simulink model "models_diff_integr"  (R2017a)
settings: Solver=VariableStepAuto  StartTime=0.0  StopTime=Time  RelTol=1e-3
undefined symbols (not defined in the file or in its folder): coeff, coeff_integrator, ts
settings Model: FPTShortcutValueString='{{},{''BaselineRun'',1,1,1,''BaselineRun'','''',{},''M'',''D'',''''}}'  Creator=kavru  LastModifiedBy=kavru
settings DataIOCC: ReturnWorkspaceOutputs=on
settings DebuggingCC: SignalRangeChecking=warning  SFMachineParentedDataDiag=error
settings SFSimCC: SimUseLocalCustomCode=on
settings RTWCC: RTWUseLocalCustomCode=on

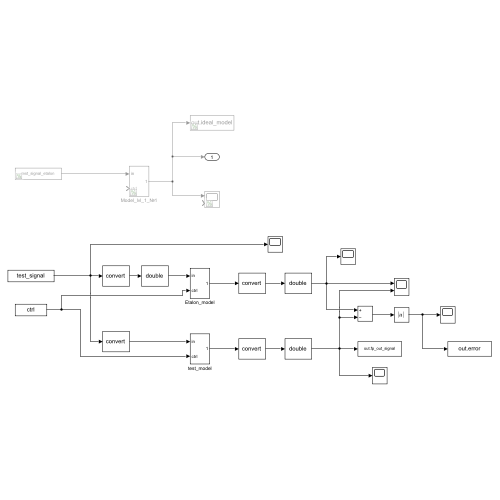
[thumbnail: Simulink's stored preview of the top-level diagram]
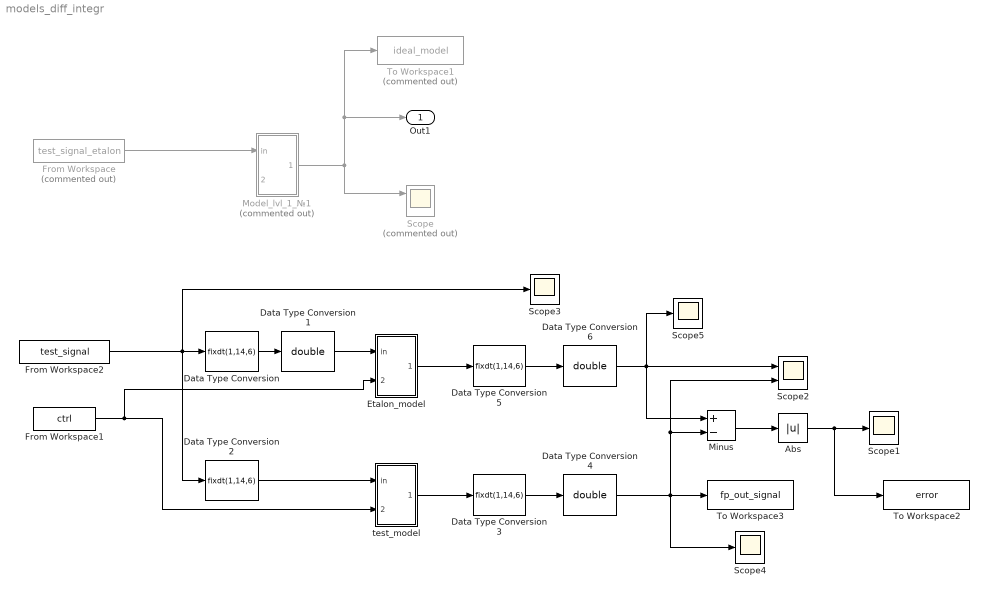
== system models_diff_integr ==
  Abs : Abs
  Data Type Conversion{,2..3,5} (4 alike) : DataTypeConversion  OutDataTypeStr=fixdt(1,14,6)  RndMeth=Nearest
  Data Type Conversion1 : DataTypeConversion  OutDataTypeStr=double
  Data Type Conversion4 : DataTypeConversion  OutDataTypeStr=double
  Data Type Conversion6 : DataTypeConversion  OutDataTypeStr=double
  Etalon_model : Subsystem
  From Workspace : FromWorkspace  Commented=on  VariableName=test_signal_etalon  OutDataTypeStr=double  SampleTime=ts
  From Workspace1 : FromWorkspace  VariableName=ctrl  SampleTime=ts
  From Workspace2 : FromWorkspace  VariableName=test_signal  OutDataTypeStr=double  SampleTime=ts
  Minus : Sum  Inputs=+-
  Model_lvl_1_№1 : Subsystem  Commented=on
  Scope : Scope  Commented=on  NumInputPorts=2
  Scope{1,3..5} (4 alike) : Scope
  Scope2 : Scope  NumInputPorts=2
  To Workspace1 : ToWorkspace  Commented=on  VariableName=ideal_model  SaveFormat=Timeseries  SampleTime=-1
  To Workspace2 : ToWorkspace  VariableName=error  SaveFormat=Timeseries  SampleTime=-1
  To Workspace3 : ToWorkspace  VariableName=fp_out_signal  SaveFormat=Timeseries  SampleTime=-1
  test_model : Subsystem
  Out1 : Outport
  wires:
  From Workspace/1 -> Model_lvl_1_№1/1(in)
  Model_lvl_1_№1/1(Out1) -> To Workspace1/1, Out1/1, Scope/1
  From Workspace2/1 -> Data Type Conversion2/1, Data Type Conversion/1, Scope3/1
  Minus/1 -> Abs/1
  Abs/1 -> Scope1/1, To Workspace2/1
  Data Type Conversion3/1 -> Data Type Conversion4/1
  Data Type Conversion4/1 -> To Workspace3/1, Minus/2, Scope2/2, Scope4/1
  Data Type Conversion6/1 -> Scope2/1, Minus/1, Scope5/1
  Data Type Conversion5/1 -> Data Type Conversion6/1
  From Workspace1/1 -> Etalon_model/2(ctrl), test_model/2(ctrl)
  test_model/1(Out1) -> Data Type Conversion3/1
  Etalon_model/1(Out1) -> Data Type Conversion5/1
  Data Type Conversion1/1 -> Etalon_model/1(in)
  Data Type Conversion2/1 -> test_model/1(in)
  Data Type Conversion/1 -> Data Type Conversion1/1

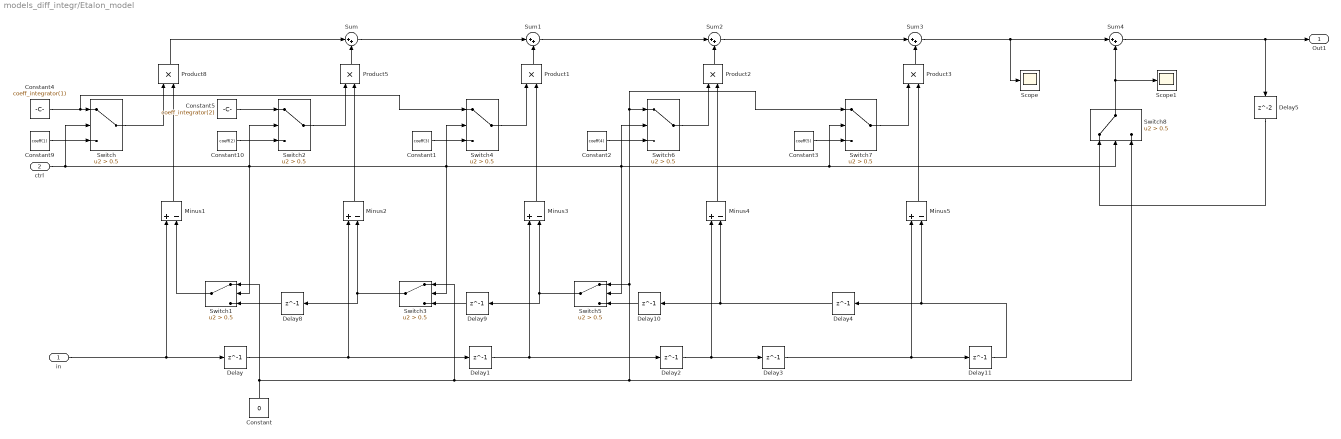
== system models_diff_integr/Etalon_model ==
  in : Inport
  ctrl : Inport  Port=2
  Constant : Constant  Value=0
  Constant1 : Constant  Value=coeff(3)
  Constant10 : Constant  Value=coeff(2)
  Constant2 : Constant  Value=coeff(4)
  Constant3 : Constant  Value=coeff(5)
  Constant4 : Constant  Value=coeff_integrator(1)
  Constant5 : Constant  Value=coeff_integrator(2)
  Constant9 : Constant  Value=coeff(1)
  Delay{,1..4,8..11} (9 alike) : Delay  DelayLength=1
  Delay5 : Delay
  Minus{1..5} (5 alike) : Sum  Inputs=+-  RndMeth=Nearest
  Product{1..3,5,8} (5 alike) : Product  RndMeth=Nearest
  Scope : Scope
  Scope1 : Scope
  Sum{,1..4} (5 alike) : Sum  Inputs=|++  RndMeth=Nearest
  Switch{,1..7} (8 alike) : Switch  Criteria=u2 > Threshold  Threshold=0.5
  Switch8 : Switch  Criteria=u2 > Threshold  Threshold=0.5  RndMeth=Nearest
  Out1 : Outport
  wires:
  Switch4/1 -> Product1/1
  Minus5/1 -> Product3/2
  Switch2/1 -> Product5/1
  Switch7/1 -> Product3/1
  Constant3/1 -> Switch7/3
  Sum1/1 -> Sum2/1
  Constant4/1 -> Switch4/1, Switch/1
  ctrl/1 -> Switch/2, Switch1/2, Switch7/2, Switch8/2, Switch6/2, Switch5/2, Switch3/2, Switch4/2, Switch2/2
  Minus4/1 -> Product2/2
  Constant10/1 -> Switch2/3
  Switch6/1 -> Product2/1
  Constant2/1 -> Switch6/3
  Sum4/1 -> Out1/1, Delay5/1
  Delay4/1 -> Minus4/2, Delay10/1
  Constant1/1 -> Switch4/3
  Delay/1 -> Delay1/1, Minus2/1
  Constant9/1 -> Switch/3
  Minus2/1 -> Product5/2
  Switch8/1 -> Scope1/1, Sum4/2
  Product5/1 -> Sum/2
  Product8/1 -> Sum/1
  Switch3/1 -> Delay8/1, Minus2/2
  Delay9/1 -> Switch3/3
  Sum3/1 -> Scope/1, Sum4/1
  Switch/1 -> Product8/1
  Constant/1 -> Switch1/1, Switch3/1, Switch6/1, Switch7/1, Switch5/1, Switch8/3
  Minus1/1 -> Product8/2
  Product3/1 -> Sum3/2
  Product1/1 -> Sum1/2
  Product2/1 -> Sum2/2
  Delay2/1 -> Delay3/1, Minus4/1
  Delay8/1 -> Switch1/3
  Delay1/1 -> Delay2/1, Minus3/1
  Sum/1 -> Sum1/1
  Switch5/1 -> Delay9/1, Minus3/2
  Minus3/1 -> Product1/2
  Delay11/1 -> Minus5/2, Delay4/1
  Switch1/1 -> Minus1/2
  Sum2/1 -> Sum3/1
  Delay3/1 -> Delay11/1, Minus5/1
  Delay10/1 -> Switch5/3
  in/1 -> Minus1/1, Delay/1
  Delay5/1 -> Switch8/1
  Constant5/1 -> Switch2/1

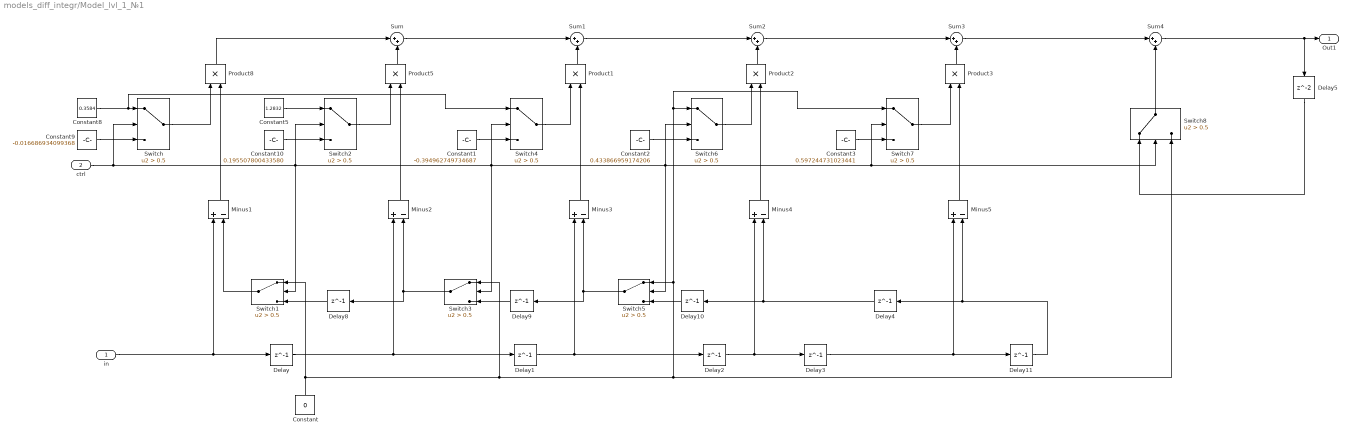
== system models_diff_integr/Model_lvl_1_№1 ==
  in : Inport
  ctrl : Inport  Port=2
  Constant : Constant  Value=0
  Constant1 : Constant  Value=-0.394962749734687
  Constant10 : Constant  Value=0.195507800433580
  Constant2 : Constant  Value=0.433866959174206
  Constant3 : Constant  Value=0.597244731023441
  Constant5 : Constant  Value=1.2832
  Constant8 : Constant  Value=0.3584
  Constant9 : Constant  Value=-0.016686934099368
  Delay{,1..4,8..11} (9 alike) : Delay  DelayLength=1
  Delay5 : Delay
  Minus{1..5} (5 alike) : Sum  Inputs=+-
  Product{1..3,5,8} (5 alike) : Product
  Sum{,1..4} (5 alike) : Sum  Inputs=|++
  Switch{,1..8} (9 alike) : Switch  Criteria=u2 > Threshold  Threshold=0.5
  Out1 : Outport
  wires:
  Delay2/1 -> Delay3/1, Minus4/1
  Sum1/1 -> Sum2/1
  Delay4/1 -> Minus4/2, Delay10/1
  Sum2/1 -> Sum3/1
  Delay3/1 -> Delay11/1, Minus5/1
  Delay1/1 -> Delay2/1, Minus3/1
  Delay11/1 -> Minus5/2, Delay4/1
  Sum/1 -> Sum1/1
  Delay/1 -> Delay1/1, Minus2/1
  in/1 -> Delay/1, Minus1/1
  Product5/1 -> Sum/2
  Product1/1 -> Sum1/2
  Product2/1 -> Sum2/2
  Product3/1 -> Sum3/2
  ctrl/1 -> Switch/2, Switch1/2, Switch7/2, Switch8/2, Switch6/2, Switch5/2, Switch3/2, Switch4/2, Switch2/2
  Sum3/1 -> Sum4/1
  Sum4/1 -> Out1/1, Delay5/1
  Switch8/1 -> Sum4/2
  Delay5/1 -> Switch8/1
  Product8/1 -> Sum/1
  Constant8/1 -> Switch4/1, Switch/1
  Constant9/1 -> Switch/3
  Switch/1 -> Product8/1
  Delay8/1 -> Switch1/3
  Constant/1 -> Switch1/1, Switch3/1, Switch6/1, Switch7/1, Switch5/1, Switch8/3
  Switch1/1 -> Minus1/2
  Minus1/1 -> Product8/2
  Constant5/1 -> Switch2/1
  Constant10/1 -> Switch2/3
  Switch2/1 -> Product5/1
  Minus2/1 -> Product5/2
  Switch3/1 -> Delay8/1, Minus2/2
  Delay9/1 -> Switch3/3
  Switch4/1 -> Product1/1
  Constant1/1 -> Switch4/3
  Minus3/1 -> Product1/2
  Delay10/1 -> Switch5/3
  Switch5/1 -> Delay9/1, Minus3/2
  Constant2/1 -> Switch6/3
  Switch6/1 -> Product2/1
  Minus4/1 -> Product2/2
  Constant3/1 -> Switch7/3
  Minus5/1 -> Product3/2
  Switch7/1 -> Product3/1

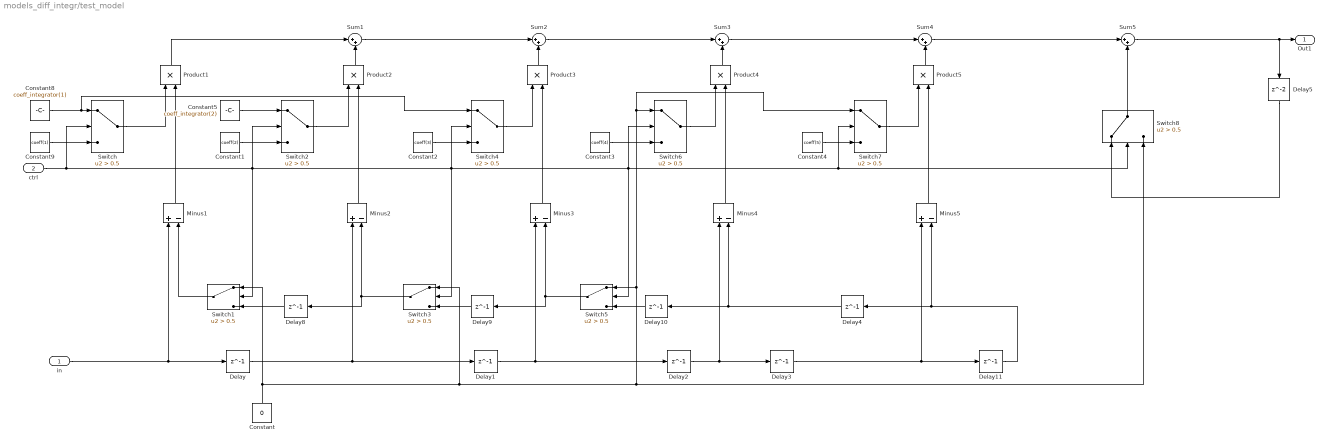
== system models_diff_integr/test_model ==
  in : Inport
  ctrl : Inport  Port=2
  Constant : Constant  Value=0
  Constant1 : Constant  Value=coeff(2)
  Constant2 : Constant  Value=coeff(3)
  Constant3 : Constant  Value=coeff(4)
  Constant4 : Constant  Value=coeff(5)
  Constant5 : Constant  Value=coeff_integrator(2)
  Constant8 : Constant  Value=coeff_integrator(1)
  Constant9 : Constant  Value=coeff(1)
  Delay{,1..4,8..11} (9 alike) : Delay  DelayLength=1
  Delay5 : Delay
  Minus{1..5} (5 alike) : Sum  Inputs=+-  AccumDataTypeStr=fixdt(1,15,6)  OutDataTypeStr=fixdt(1,15,6)  RndMeth=Nearest
  Product1 : Product  OutDataTypeStr=fixdt(1,18,12)  RndMeth=Nearest
  Product2 : Product  OutDataTypeStr=fixdt(1,19,11)  RndMeth=Nearest
  Product3 : Product  OutDataTypeStr=fixdt(1,20,12)  RndMeth=Nearest
  Product4 : Product  OutDataTypeStr=fixdt(1,14,6)  RndMeth=Nearest
  Product5 : Product  OutDataTypeStr=fixdt(1,14,6)  RndMeth=Nearest
  Sum{1..5} (5 alike) : Sum  Inputs=|++  OutDataTypeStr=fixdt(1,20,12)  RndMeth=Nearest
  Switch{,1..8} (9 alike) : Switch  Criteria=u2 > Threshold  Threshold=0.5
  Out1 : Outport
  wires:
  Minus3/1 -> Product3/2
  Switch4/1 -> Product3/1
  Constant/1 -> Switch1/1, Switch3/1, Switch6/1, Switch7/1, Switch5/1, Switch8/3
  Product3/1 -> Sum2/2
  Constant2/1 -> Switch4/3
  Constant8/1 -> Switch4/1, Switch/1
  Delay/1 -> Minus2/1, Delay1/1
  Sum2/1 -> Sum3/1
  Product4/1 -> Sum3/2
  Sum3/1 -> Sum4/1
  Constant4/1 -> Switch7/3
  Delay4/1 -> Minus4/2, Delay10/1
  Switch6/1 -> Product4/1
  Switch3/1 -> Minus2/2, Delay8/1
  Switch2/1 -> Product2/1
  Product2/1 -> Sum1/2
  Delay11/1 -> Minus5/2, Delay4/1
  Delay5/1 -> Switch8/1
  ctrl/1 -> Switch/2, Switch1/2, Switch7/2, Switch8/2, Switch6/2, Switch5/2, Switch3/2, Switch4/2, Switch2/2
  in/1 -> Delay/1, Minus1/1
  Minus1/1 -> Product1/2
  Constant3/1 -> Switch6/3
  Switch/1 -> Product1/1
  Delay3/1 -> Minus5/1, Delay11/1
  Product1/1 -> Sum1/1
  Constant1/1 -> Switch2/3
  Minus2/1 -> Product2/2
  Switch1/1 -> Minus1/2
  Delay9/1 -> Switch3/3
  Switch5/1 -> Minus3/2, Delay9/1
  Constant9/1 -> Switch/3
  Delay2/1 -> Minus4/1, Delay3/1
  Delay8/1 -> Switch1/3
  Minus5/1 -> Product5/2
  Delay10/1 -> Switch5/3
  Minus4/1 -> Product4/2
  Switch7/1 -> Product5/1
  Constant5/1 -> Switch2/1
  Delay1/1 -> Minus3/1, Delay2/1
  Sum1/1 -> Sum2/1
  Product5/1 -> Sum4/2
  Sum4/1 -> Sum5/1
  Switch8/1 -> Sum5/2
  Sum5/1 -> Delay5/1, Out1/1
